simulink subsystem "HighLevelController"  (R2023a)
settings: Solver=VariableStepAuto  StartTime=0.0  StopTime=10.0  RelTol=1e-3
settings Model: Creator=stude  LastModifiedBy=mehra

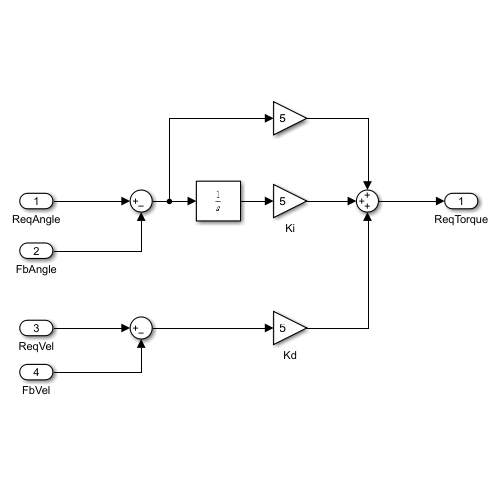
[thumbnail: Simulink's stored preview of the top-level diagram]
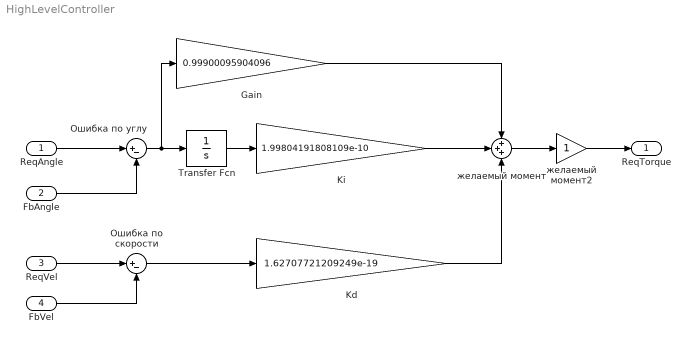
== system HighLevelController ==
  ReqAngle : Inport
  FbAngle : Inport  Port=2
  ReqVel : Inport  Port=3
  FbVel : Inport  Port=4
  Gain : Gain  Gain=0.99900095904096
  Kd : Gain  Gain=1.62707721209249e-19
  Ki : Gain  Gain=1.99804191808109e-10
  Transfer Fcn : TransferFcn  Denominator=[1 0]
  Ошибка по скорости : Sum  Inputs=|+-
  Ошибка по углу : Sum  Inputs=|+-
  желаемый момент : Sum  Inputs=+++
  желаемый момент2 : Gain
  ReqTorque : Outport
  wires:
  FbAngle/1 -> Ошибка по углу/2
  FbVel/1 -> Ошибка по скорости/2
  ReqAngle/1 -> Ошибка по углу/1
  Ki/1 -> желаемый момент/2
  ReqVel/1 -> Ошибка по скорости/1
  Kd/1 -> желаемый момент/3
  Gain/1 -> желаемый момент/1
  желаемый момент/1 -> желаемый момент2/1
  Transfer Fcn/1 -> Ki/1
  Ошибка по скорости/1 -> Kd/1
  Ошибка по углу/1 -> Gain/1, Transfer Fcn/1
  желаемый момент2/1 -> ReqTorque/1
